simulink model "pmsm_foc_qep_lvmc_template"  (R2022b)
settings: Solver=FixedStepDiscrete  StartTime=0.0  StopTime=10.0  FixedStep=50e-6  RelTol=1e-3  EnableMultiTasking=on
values from neighbouring files (symbols this model uses):
  PI_params = mcb.internal.SetControllerParameters(pmsm,inverter,PU_System,T_pwm,Ts,Ts_speed)    [mcb_pmsm_foc_qep_dsPIC33_data.m]
  PU_System = mcb_SetPUSystem(pmsm,inverter)    [mcb_pmsm_foc_qep_dsPIC33_data.m]
  PWM_frequency = 20e3    (= 20000)    [mcb_pmsm_foc_qep_dsPIC33_data.m]
  Ts = T_pwm    (= 5e-05)    [mcb_pmsm_foc_qep_dsPIC33_data.m]
  Ts_speed = 30*Ts    (= 0.0015)    [mcb_pmsm_foc_qep_dsPIC33_data.m]
undefined symbols (not defined in the file or in its folder): A0, A4, AN0, AN1, B0, B2, C12, C13, C14, C7, D11, D12, D13, D14, D5, D6, D7, DiscIntNeverNeededParam, inverter, Max, MaxPer, ms, NumBits1, NumBits2, P20, P32, P55, P60, P61, P62, P69, P70, P71, P75, P76, P77, P78, Pin, pmsm, PWM1max, Resol, s, us
libraries: simulink x28, MCHP_Blockset x22, mcbcontrolslib x9, slpidlib x3, mcbpositiondecoderlib x3, mcbplantlib x1, autolibpmsmexterior x1
(part 4 of 4)

== system pmsm_foc_qep_lvmc_template/Inverter and Motor/Simulation/Inverter ==
  Duty_abc : Inport
  Average-Value Inverter : mcbplantlib/Average-Value Inverter
  Constant2 : Constant  Value=inverter.V_dc  OutDataTypeStr=single  SampleTime=-1
  Data Type Conversion1 : DataTypeConversion  OutDataTypeStr=single  RndMeth=Simplest  SaturateOnIntegerOverflow=off
  Vabc : Outport  VectorParamsAs1DForOutWhenUnconnected=off
  wires:
  Average-Value Inverter/1 -> Vabc/1
  Data Type Conversion1/1 -> Average-Value Inverter/1
  Duty_abc/1 -> Data Type Conversion1/1
  Constant2/1 -> Average-Value Inverter/2

== system pmsm_foc_qep_lvmc_template/Inverter and Motor/Simulation/Load_Profile (Torque) ==
  Data Type Conversion : DataTypeConversion  OutDataTypeStr=single  SaturateOnIntegerOverflow=off  RndMeth=Floor
  IIR Filter : mcbcontrolslib/IIR Filter  VariantControl=Low Pass Filter  VariantSelect=Low-pass  Filter_constant=0.01  advancedSettings=off  Ts=50e-6  cutOff_freq=32.1525
  Step : Step  Time=8  Before=0.05 * pmsm.T_rated  After=0.5 * pmsm.T_rated
  Load_Trq : Outport  VectorParamsAs1DForOutWhenUnconnected=off
  wires:
  IIR Filter/1 -> Load_Trq/1
  Data Type Conversion/1 -> IIR Filter/1
  Step/1 -> Data Type Conversion/1

== system pmsm_foc_qep_lvmc_template/Inverter and Motor/Simulation/Sensor_Measurements ==
  note: Delays
  note: Scaling
  Info : Inport
  PhaseCurr : Inport  Port=2
  Bus Selector : BusSelector  OutputSignals=MtrPos
  Data Type Conversion2 : DataTypeConversion  OutDataTypeStr=single  RndMeth=Simplest  SaturateOnIntegerOverflow=off
  Data Type Conversion4 : DataTypeConversion  OutDataTypeStr=single  RndMeth=Simplest  SaturateOnIntegerOverflow=off
  Delay1 : Delay  DelayLength=PI_params.delay_Currents
  Delay2 : Delay  DelayLength=PI_params.delay_Position
  "Get_PU " : Subsystem
  Get_QEP_Counts : Gain  Gain=pmsm.QEPSlits  OutDataTypeStr=uint16  RndMeth=Simplest
  Inverting OpAmp : Gain  Gain=1/PU_System.I_base  OutDataTypeStr=dataType  RndMeth=Simplest
  Selector : Selector  InputPortWidth=3  IndexOptions=Index vector (dialog)  Indices=[1 2]  OutputSizes=1
  Iab_fb : Outport  VectorParamsAs1DForOutWhenUnconnected=off
  Pos_fb : Outport  Port=2  VectorParamsAs1DForOutWhenUnconnected=off
  wires:
  Selector/1 -> Inverting OpAmp/1
  Delay2/1 -> "Get_PU "/1(rad)  "Theta_m"
  Data Type Conversion2/1 -> Delay2/1  "Theta_m"
  Bus Selector/1 -> Data Type Conversion2/1  "<MtrPos>"
  Info/1 -> Bus Selector/1
  PhaseCurr/1 -> Data Type Conversion4/1
  Data Type Conversion4/1 -> Delay1/1
  Delay1/1 -> Selector/1  "Iab_fb"
  "Get_PU "/1(PU) -> Get_QEP_Counts/1
  Inverting OpAmp/1 -> Iab_fb/1
  Get_QEP_Counts/1 -> Pos_fb/1

== system pmsm_foc_qep_lvmc_template/Speed Control/Enable Switch/Codegen ==

== system pmsm_foc_qep_lvmc_template/Speed Control/Enable Switch/Sim ==
  Constant : Constant  OutDataTypeStr=Inherit: Inherit via back propagation
  Data Store Write : DataStoreWrite  DataStoreName=Enable  IndexOptions=Index vector (dialog)  Indices=1  OutputSizes=1
  wires:
  Constant/1 -> Data Store Write/1

== system pmsm_foc_qep_lvmc_template/Current Control/Closed Loop Control/Current_Controllers/PI_Controller_Id ==
  I_ref : Inport
  I_fb : Inport  Port=2
  AND : Logic  IconShape=distinctive  AllPortsSameDT=off  OutDataTypeStr=boolean
  Data Store Read1 : DataStoreRead  DataStoreName=EnableFOC  IndexOptions=Index vector (dialog)  Indices=1  OutputSizes=1
  Data Store Read2 : DataStoreRead  DataStoreName=Enable  IndexOptions=Index vector (dialog)  Indices=1  OutputSizes=1
  Discrete PI Controller with anti-windup & reset : slpidlib/PID Controller  Controller=PI  Form=Parallel  TimeDomain=Discrete-time  UseExternalTs=off  SampleTime=-1  IntegratorMethod=Forward Euler  FilterMethod=Forward Euler  ControllerParametersSource=external  P=1  I=1  UseKiTs=on  D=0  N=100  UseFilter=on  TunerSelectOption=Transfer Function Based (PID Tuner App)  InitialConditionSource=external  InitialConditionForIntegrator=0  InitialConditionForFilter=0  DifferentiatorICPrevScaledInput=0  ExternalReset=level  TrackingMode=off  Kt=1  LimitOutput=on  SatLimitsSource=internal  UpperSaturationLimit=1  LowerSaturationLimit=-1  LinearizeAsGain=on  AntiWindupMode=clamping  Kb=1  LimitIntegrator=off  UpperIntegratorSaturationLimit=inf  LowerIntegratorSaturationLimit=-inf  RndMeth=Simplest  POutMin=[]  POutMax=[]  IOutMin=[]  IOutMax=[]  DOutMin=[]  DOutMax=[]  NOutMin=[]  NOutMax=[]  SumOutMin=[]  SumOutMax=[]  SaturationOutDataTypeStr=Inherit: Inherit via back propagation  SaturationOutMin=[]  SaturationOutMax=[]  PParamMin=[]  PParamMax=[]  IParamMin=[]  IParamMax=[]  DParamMin=[]  DParamMax=[]  NParamMin=[]  NParamMax=[]  KbParamMin=[]  KbParamMax=[]  KtParamMin=[]  KtParamMax=[]  KbOutMin=[]  KbOutMax=[]  KtOutMin=[]  KtOutMax=[]  IntegratorOutMin=[]  IntegratorOutMax=[]  FilterOutMin=[]  FilterOutMax=[]  SumI1OutMin=[]  SumI1OutMax=[]  SumI2OutMin=[]  SumI2OutMax=[]  SumI3OutMin=[]  SumI3OutMax=[]  SumI4OutMin=[]  SumI4OutMax=[]  SumDOutMin=[]  SumDOutMax=[]  DifferentiatorOutMin=[]  DifferentiatorOutMax=[]  FilterDiffOutCoefMin=[]  FilterDiffOutCoefMax=[]  ReciprocalOutMin=[]  ReciprocalOutMax=[]  SumDenOutMin=[]  SumDenOutMax=[]  SumNumOutMin=[]  SumNumOutMax=[]  DivideOutMin=[]  DivideOutMax=[]  UdiffTsProdOutMin=[]  UdiffTsProdOutMax=[]  NTsProdOutMin=[]  NTsProdOutMax=[]  UintegralTsProdOutMin=[]  UintegralTsProdOutMax=[]  UngainTsProdOutMin=[]  UngainTsProdOutMax=[]  ClampingZeroOutDataTypeStr=Inherit: Inherit via back propagation  ClampingZeroOutMin=[]  ClampingZeroOutMax=[]  FilterDenConstantOutDataTypeStr=Inherit: Inherit via back propagation  FilterDenConstantOutMin=[]  FilterDenConstantOutMax=[]  PCopyOutDataTypeStr=Inherit: Inherit via back propagation  PCopyOutMin=[]  PCopyOutMax=[]  NCopyOutDataTypeStr=Inherit: Inherit via back propagation  NCopyOutMin=[]  NCopyOutMax=[]  IntegratorContinuousStateAttributes=''  IntegratorStateMustResolveToSignalObject=off  IntegratorRTWStateStorageClass=Auto  FilterContinuousStateAttributes=''  FilterStateMustResolveToSignalObject=off  FilterRTWStateStorageClass=Auto  ParallelPVariant=ExternalParameters  IdealPVariant=Disabled  IVariant=ExternalParameters  DVariant=Disabled  IntegratorVariant=Discrete  SatVariant=Enabled  AWVariant=DiscClampingParallel  PCopyVariant=Disabled  TRVariant=Disabled  FdbkBlocksVariant=Forward  IdealPFdbkVariant=Disabled  SatFdbkVariant=Disabled  DerivativeFilterVariant=Disabled  NVariant=Disabled  NCopyVariant=Disabled_SignalSpec  FilterICVariant=Disabled  IntegratorICVariant=ExternalICs  ExternalResetVariant=ExternalReset  TRSumVariant=Passthrough  SumFdbkVariant=Disabled  SumVariant=Sum_PI  TsampFilterVariant=InternalTs  TsampNgainVariant=Passthrough  TsampIntegralVariant=Passthrough  ExternalSaturationOutDataTypeStr=Inherit: Same as second input
  Ki : Constant  Value=PI_params.Ki_i*Ts/2  OutDataTypeStr=dataType  SampleTime=-1
  Ki1 : Constant  Value=0  OutDataTypeStr=dataType  SampleTime=-1
  Kp : Constant  Value=PI_params.Kp_i/2  OutDataTypeStr=dataType2  SampleTime=-1
  Logical Operator : Logic  Operator=NOT  IconShape=distinctive  AllPortsSameDT=off  OutDataTypeStr=boolean
  Sum : Sum  Inputs=|+-  OutDataTypeStr=Inherit: Same as first input
  V_ref : Outport  VectorParamsAs1DForOutWhenUnconnected=off
  wires:
  I_ref/1 -> Sum/1
  I_fb/1 -> Sum/2
  AND/1 -> Logical Operator/1
  Discrete PI Controller with anti-windup & reset/1 -> V_ref/1
  Sum/1 -> Discrete PI Controller with anti-windup & reset/1
  Kp/1 -> Discrete PI Controller with anti-windup & reset/2
  Ki/1 -> Discrete PI Controller with anti-windup & reset/3
  Logical Operator/1 -> Discrete PI Controller with anti-windup & reset/4
  Ki1/1 -> Discrete PI Controller with anti-windup & reset/5
  Data Store Read1/1 -> AND/1
  Data Store Read2/1 -> AND/2

== system pmsm_foc_qep_lvmc_template/Current Control/Closed Loop Control/Current_Controllers/PI_Controller_Iq ==
  I_ref : Inport
  I_fb : Inport  Port=2
  AND : Logic  IconShape=distinctive  AllPortsSameDT=off  OutDataTypeStr=boolean
  Data Store Read1 : DataStoreRead  DataStoreName=EnableFOC  IndexOptions=Index vector (dialog)  Indices=1  OutputSizes=1
  Data Store Read2 : DataStoreRead  DataStoreName=Enable  IndexOptions=Index vector (dialog)  Indices=1  OutputSizes=1
  Discrete PI Controller with anti-windup & reset : slpidlib/PID Controller  Controller=PI  Form=Parallel  TimeDomain=Discrete-time  UseExternalTs=off  SampleTime=-1  IntegratorMethod=Forward Euler  FilterMethod=Forward Euler  ControllerParametersSource=external  P=1  I=1  UseKiTs=on  D=0  N=100  UseFilter=on  TunerSelectOption=Transfer Function Based (PID Tuner App)  InitialConditionSource=external  InitialConditionForIntegrator=0  InitialConditionForFilter=0  DifferentiatorICPrevScaledInput=0  ExternalReset=level  TrackingMode=off  Kt=1  LimitOutput=on  SatLimitsSource=internal  UpperSaturationLimit=1  LowerSaturationLimit=-1  LinearizeAsGain=on  AntiWindupMode=clamping  Kb=1  LimitIntegrator=off  UpperIntegratorSaturationLimit=inf  LowerIntegratorSaturationLimit=-inf  RndMeth=Simplest  POutMin=[]  POutMax=[]  IOutMin=[]  IOutMax=[]  DOutMin=[]  DOutMax=[]  NOutMin=[]  NOutMax=[]  SumOutMin=[]  SumOutMax=[]  SaturationOutDataTypeStr=Inherit: Inherit via back propagation  SaturationOutMin=[]  SaturationOutMax=[]  PParamMin=[]  PParamMax=[]  IParamMin=[]  IParamMax=[]  DParamMin=[]  DParamMax=[]  NParamMin=[]  NParamMax=[]  KbParamMin=[]  KbParamMax=[]  KtParamMin=[]  KtParamMax=[]  KbOutMin=[]  KbOutMax=[]  KtOutMin=[]  KtOutMax=[]  IntegratorOutMin=[]  IntegratorOutMax=[]  FilterOutMin=[]  FilterOutMax=[]  SumI1OutMin=[]  SumI1OutMax=[]  SumI2OutMin=[]  SumI2OutMax=[]  SumI3OutMin=[]  SumI3OutMax=[]  SumI4OutMin=[]  SumI4OutMax=[]  SumDOutMin=[]  SumDOutMax=[]  DifferentiatorOutMin=[]  DifferentiatorOutMax=[]  FilterDiffOutCoefMin=[]  FilterDiffOutCoefMax=[]  ReciprocalOutMin=[]  ReciprocalOutMax=[]  SumDenOutMin=[]  SumDenOutMax=[]  SumNumOutMin=[]  SumNumOutMax=[]  DivideOutMin=[]  DivideOutMax=[]  UdiffTsProdOutMin=[]  UdiffTsProdOutMax=[]  NTsProdOutMin=[]  NTsProdOutMax=[]  UintegralTsProdOutMin=[]  UintegralTsProdOutMax=[]  UngainTsProdOutMin=[]  UngainTsProdOutMax=[]  ClampingZeroOutDataTypeStr=Inherit: Inherit via back propagation  ClampingZeroOutMin=[]  ClampingZeroOutMax=[]  FilterDenConstantOutDataTypeStr=Inherit: Inherit via back propagation  FilterDenConstantOutMin=[]  FilterDenConstantOutMax=[]  PCopyOutDataTypeStr=Inherit: Inherit via back propagation  PCopyOutMin=[]  PCopyOutMax=[]  NCopyOutDataTypeStr=Inherit: Inherit via back propagation  NCopyOutMin=[]  NCopyOutMax=[]  IntegratorContinuousStateAttributes=''  IntegratorStateMustResolveToSignalObject=off  IntegratorRTWStateStorageClass=Auto  FilterContinuousStateAttributes=''  FilterStateMustResolveToSignalObject=off  FilterRTWStateStorageClass=Auto  ParallelPVariant=ExternalParameters  IdealPVariant=Disabled  IVariant=ExternalParameters  DVariant=Disabled  IntegratorVariant=Discrete  SatVariant=Enabled  AWVariant=DiscClampingParallel  PCopyVariant=Disabled  TRVariant=Disabled  FdbkBlocksVariant=Forward  IdealPFdbkVariant=Disabled  SatFdbkVariant=Disabled  DerivativeFilterVariant=Disabled  NVariant=Disabled  NCopyVariant=Disabled_SignalSpec  FilterICVariant=Disabled  IntegratorICVariant=ExternalICs  ExternalResetVariant=ExternalReset  TRSumVariant=Passthrough  SumFdbkVariant=Disabled  SumVariant=Sum_PI  TsampFilterVariant=InternalTs  TsampNgainVariant=Passthrough  TsampIntegralVariant=Passthrough  ExternalSaturationOutDataTypeStr=Inherit: Same as second input
  Ki : Constant  Value=PI_params.Ki_i*Ts/2  OutDataTypeStr=dataType  SampleTime=-1
  Kp : Constant  Value=PI_params.Kp_i/2  OutDataTypeStr=dataType2  SampleTime=-1
  Kp1 : Constant  Value=0  OutDataTypeStr=dataType  SampleTime=-1
  Logical Operator : Logic  Operator=NOT  IconShape=distinctive  AllPortsSameDT=off  OutDataTypeStr=boolean
  Sum : Sum  Inputs=|+-  OutDataTypeStr=Inherit: Same as first input
  V_ref : Outport  VectorParamsAs1DForOutWhenUnconnected=off
  wires:
  Discrete PI Controller with anti-windup & reset/1 -> V_ref/1
  I_fb/1 -> Sum/2
  I_ref/1 -> Sum/1
  Kp/1 -> Discrete PI Controller with anti-windup & reset/2
  Sum/1 -> Discrete PI Controller with anti-windup & reset/1
  Ki/1 -> Discrete PI Controller with anti-windup & reset/3
  Logical Operator/1 -> Discrete PI Controller with anti-windup & reset/4
  Kp1/1 -> Discrete PI Controller with anti-windup & reset/5
  Data Store Read1/1 -> AND/1
  Data Store Read2/1 -> AND/2
  AND/1 -> Logical Operator/1

== system pmsm_foc_qep_lvmc_template/Current Control/Output Scaling/Mode Selector/Subsystem1 ==
  Count : Inport
  AND : Logic  IconShape=distinctive  AllPortsSameDT=off  OutDataTypeStr=boolean
  Compare To Constant : simulink/Logic and Bit Operations/Compare To Constant  relop=>=  const=3.0  OutDataTypeStr=boolean
  Compare To Constant1 : simulink/Logic and Bit Operations/Compare To Constant  relop=<  const=1  OutDataTypeStr=boolean
  Compare To Constant2 : simulink/Logic and Bit Operations/Compare To Constant  relop=<  const=2  OutDataTypeStr=boolean
  Compare To Constant3 : simulink/Logic and Bit Operations/Compare To Constant  relop=>  const=1  OutDataTypeStr=boolean
  Data Store Write : DataStoreWrite  DataStoreName=EnCurOffset  IndexOptions=Index vector (dialog)  Indices=1  OutputSizes=1
  Data Store Write1 : DataStoreWrite  DataStoreName=EnableFOC  IndexOptions=Index vector (dialog)  Indices=1  OutputSizes=1
  Data Store Write2 : DataStoreWrite  DataStoreName=EnPosOffset  IndexOptions=Index vector (dialog)  Indices=1  OutputSizes=1
  Gain : Gain  Gain=1/(2*PWM_frequency)  OutDataTypeStr=dataType2  RndMeth=Simplest
  Current Offset : Outport
  PositionOffset : Outport  Port=2
  EnClosedLoop : Outport  Port=3
  wires:
  Count/1 -> Gain/1
  Gain/1 -> Compare To Constant1/1, Compare To Constant3/1, Compare To Constant2/1, Compare To Constant/1
  Compare To Constant/1 -> Data Store Write1/1, EnClosedLoop/1
  Compare To Constant1/1 -> Data Store Write/1, Current Offset/1
  Compare To Constant2/1 -> AND/2
  Compare To Constant3/1 -> AND/1
  AND/1 -> Data Store Write2/1, PositionOffset/1

== system pmsm_foc_qep_lvmc_template/Current Control/Output Scaling/Mode Selector/Up Counter ==
  Enable : EnablePort  StatesWhenEnabling=reset
  Add1 : Sum  SaturateOnIntegerOverflow=on
  Constant : Constant  OutDataTypeStr=uint32
  Delay : Delay  DelayLength=1
  Count : Outport  InitialOutput=0
  wires:
  Delay/1 -> Add1/2
  Add1/1 -> Count/1, Delay/1
  Constant/1 -> Add1/1

== system pmsm_foc_qep_lvmc_template/Current Control/Serial Tx/UART_TX/Debug_Data ==
  Count : Inport
  Data : Inport  Port=2
  Bitwise Operator2 : simulink/Logic and Bit Operations/Bitwise Operator  logicop=AND  UseBitMask=on  BitMask=bin2dec('0000000011111111')  BitMaskRealWorld=Stored Integer
  Bitwise Operator3 : simulink/Logic and Bit Operations/Bitwise Operator  logicop=AND  UseBitMask=on  BitMask=bin2dec('0000000011111111')  BitMaskRealWorld=Stored Integer
  Data Type Conversion1 : DataTypeConversion  OutDataTypeStr=uint8  RndMeth=Simplest  SaturateOnIntegerOverflow=off
  Data Type Conversion2 : DataTypeConversion  OutDataTypeStr=uint8  RndMeth=Simplest  SaturateOnIntegerOverflow=off
  Data Type Conversion3 : DataTypeConversion  OutDataTypeStr=uint16  ConvertRealWorld=Stored Integer (SI)  RndMeth=Simplest  SaturateOnIntegerOverflow=off
  Mux : Mux  Inputs=3
  Shift Arithmetic2 : ArithShift  BitShiftNumber=8  BitShiftDirection=Right
  Data_log : Outport
  wires:
  Mux/1 -> Data_log/1
  Data/1 -> Data Type Conversion3/1
  Count/1 -> Mux/1
  Bitwise Operator2/1 -> Data Type Conversion1/1
  Shift Arithmetic2/1 -> Bitwise Operator3/1
  Bitwise Operator3/1 -> Data Type Conversion2/1
  Data Type Conversion3/1 -> Bitwise Operator2/1, Shift Arithmetic2/1
  Data Type Conversion1/1 -> Mux/2
  Data Type Conversion2/1 -> Mux/3

== system pmsm_foc_qep_lvmc_template/Current Control/Serial Tx/UART_TX/SCI_Tx ==
  Data_Log : Inport
  End : Constant  Value=hex2dec('45')  OutDataTypeStr=uint8
  Mux : Mux  Inputs=3
  Start : Constant  Value=hex2dec('53')  OutDataTypeStr=uint8
  UART Tx : MCHP_Blockset/BUS UART/UART Tx  UART_REF=1  ORDERING=None  AllOrNothing=off  SampleTime=-1  MCHP_MASTERLINK=pmsm_foc_qep_lvmc_template/BOARD dsPIC33CK LVMC/Microchip Master  NSend_Input=off  UART_String=off  NSend_Output=off
      settings: SourceProductName=MPLAB Device Blocks for Simulink
  wires:
  Mux/1 -> UART Tx/1
  Data_Log/1 -> Mux/2
  Start/1 -> Mux/1
  End/1 -> Mux/3

== system pmsm_foc_qep_lvmc_template/Inverter and Motor/Simulation/Sensor_Measurements/Get_PU  ==
  rad : Inport
  Constant2 : Constant  Value=2*pi  OutDataTypeStr=single  SampleTime=-1
  Get_PU : Gain  Gain=1/(2*pi)  OutDataTypeStr=dataType  RndMeth=Simplest
  Mod : Math  Operator=mod
  PU : Outport  VectorParamsAs1DForOutWhenUnconnected=off
  wires:
  Mod/1 -> Get_PU/1
  Constant2/1 -> Mod/2
  rad/1 -> Mod/1
  Get_PU/1 -> PU/1
